simulink library "Capacitor"  (R2020b)
settings: Solver=ode45  StartTime=0.0  StopTime=10.0  RelTol=1e-3  EnableMultiTasking=on
undefined symbols (not defined in the file): Fsw_M, L_M, QgTotal_M, RL_M, Ron_M, Vgate_M
libraries: Lib_Dyn_StateSpace_TMATS x2, Lib_PF_BusLoadDC_TMATS x1
Description:
  | Thomas Modules
settings Model: Creator=jwchapm2  LastModifiedBy=nbutler2
settings DataIOCC: LimitDataPoints=on  SaveFormat=Array  ReturnWorkspaceOutputs=off
settings OptimizationCC: ExpressionDepthLimit=2147483647  LifeSpan=inf
settings DebuggingCC: UnderspecifiedInitializationDetection=Classic  MergeDetectMultiDrivingBlocksExec=none  SolverPrmCheckMsg=warning  StateNameClashWarn=warning  SFUnexpectedBacktrackingDiag=warning  SFNoUnconditionalDefaultTransitionDiag=warning  SFExecutionAtInitializationDiag=none  ArithmeticOperatorsInVariantConditions=warning
settings HardwareCC: ProdBitPerPointer=32  ProdBitPerSizeT=32  ProdBitPerPtrDiffT=32  ProdLargestAtomicFloat=None  ProdIntDivRoundTo=Undefined  ProdEndianess=Unspecified  ProdWordSize=32  ProdHWDeviceType=32-bit Generic
settings ModelReferenceCC: PropagateSignalLabelsOutOfModel=off
settings SFSimCC: SimUseLocalCustomCode=off  CustomCodeUndefinedFunction=UseInterfaceOnly
settings RTWCC: RTWUseLocalCustomCode=off
settings CodeAppCC: StateflowObjectComments=on
settings GRTTargetCC: TargetLangStandard=C89/C90 (ANSI)
settings ConfigComp: CovMetricSettings=dw  CovSaveCumulativeToWorkspaceVar=on  CovSaveSingleToWorkspaceVar=on  CovExternalEMLEnable=off

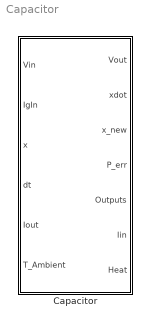
== system Capacitor ==
  Capacitor : Subsystem  mask(Capacitor){Pdis_M=1, C_M=600e-6, RC_M=1e-3, TempIn=Celsius}
      mask prompts: Pdis_M "Pdis_M - Constant Power Leaked/Dissipated, W"; C_M "C_M - Capacitor, Farads"; RC_M "RC_M - Resistance of Capacitor, Ohms"; TempIn "Input Temp Units"
      mask help: This block represents a generic capacitor energy storage element. The input current is solved for, such that the power in equals the power out.
      mask init:
      | %Get current block name
      | block = gcb;
      | 
      | %Block under the mask(T_in inport)
      | block2 = [block '/T_Ambient'];
      | 
      | %Set T_in unit parameter to correct unit.
      | switch TempIn
      |     case 1 
      |         set_param(block2,'Unit','degF');
      |     case 2
      |         set_param(block2,'Unit','degC');
      |     case 3
      |         set_param(block2,'Unit','degR');
      |     case 4
      |         set_param(block2,'Unit','K');
      | end
      mask TypeOptions TempIn: Fahrenheit | Celsius | Rankine | Kelvin
      mask DialogControl Container10 Prompt: Physical Parameters
      mask DialogControl Container11 Prompt: Temperature Units
      mask Display:
      | switch TempIn
      |     case 1
      |         port_label('input', 6, 'T_Ambient (F)');
      |     case 2
      |         port_label('input', 6, 'T_Ambient (C)');
      |     case 3
      |         port_label('input', 6, 'T_Ambient (Ra)');
      |     case 4
      |         port_label('input', 6, 'T_Ambient (K)');
      | end
      | 
      | port_label('input', 1, 'Vin');
      | port_label('input', 2, 'IgIn');
      | port_label('input', 3, 'x');
      | port_label('input', 4, 'dt');
      | port_label('input', 5, 'Idemand');
      | 
      | 
      | 
      | port_label('output', 1, 'Vout');
      | port_label('output', 2, 'xdot');
      | port_label('output', 3, 'x_new');
      | port_label('output', 4, 'P_err');
      | port_label('output', 5, 'Outputs');
      | port_label('output', 6, 'Idemanded');
      | port_label('output', 7, 'Heat');

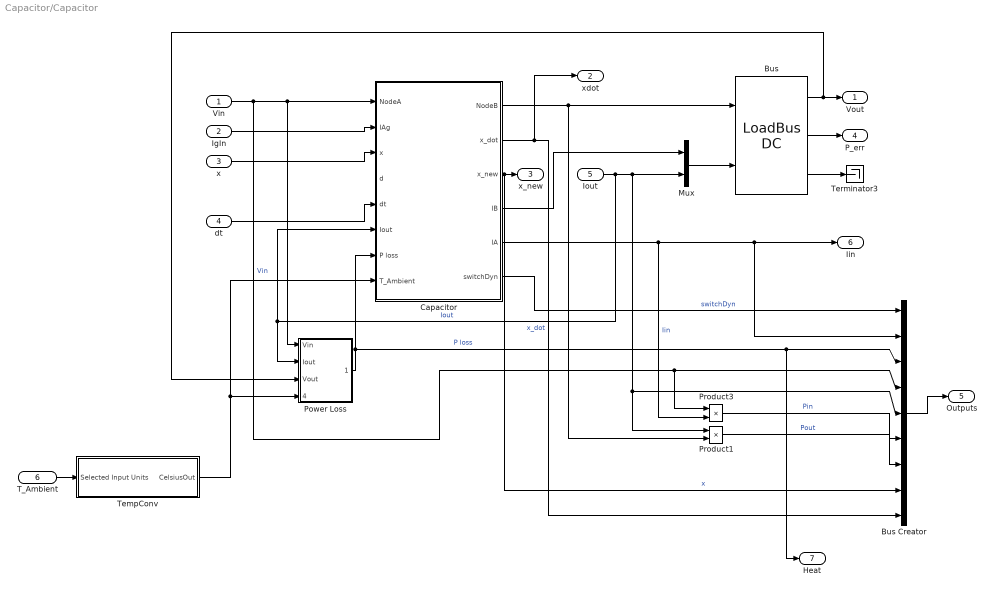
== system Capacitor/Capacitor ==
  Vin : Inport
  IgIn : Inport  Port=2
  x : Inport  Port=3
  dt : Inport  Port=4
  Iout : Inport  Port=5
  T_Ambient : Inport  Port=6  Unit=degC
  Bus : Lib_PF_BusLoadDC_TMATS/LoadBus DC  PeInEN_M=off  P_M=-Pdis_M  BlkNm_M=double(gcb)
  Bus Creator : BusCreator  Inputs=9
  Capacitor : Subsystem
      mask Display:
      | fprintf('Capacitor')
      | 
      | port_label('input',1,'VA')
      | port_label('input',2,'IAg')
      | port_label('input',3,'x')
      | port_label('input',4,'d')
      | port_label('input',5,'dt')
      | port_label('input',6,'Iout')
      | port_label('input',7,'Ploss')
      | 
      | 
      | port_label('output',1,'VB')
      | port_label('output',2,'x_dot')
      | port_label('output',3,'x_new')
      | port_label('output',4,'IB')
      | port_label('output',5,'IA')
      | port_label('output',6,'switchDyn')
  Mux : Mux  Inputs=2
  "Power Loss " : Subsystem
  Product1 : Product
  Product3 : Product
  "TempConv " : Subsystem  AncestorBlock=Lib_PB_MultiLevelInverter_TMATS/HiFiInverter/TempConv
      mask DialogControl DescTextVar Prompt: Temperature Unit Converter
  Terminator3 : Terminator
  Vout : Outport  VectorParamsAs1DForOutWhenUnconnected=off
  xdot : Outport  Port=2  VectorParamsAs1DForOutWhenUnconnected=off
  x_new : Outport  Port=3  VectorParamsAs1DForOutWhenUnconnected=off
  P_err : Outport  Port=4  VectorParamsAs1DForOutWhenUnconnected=off
  Outputs : Outport  Port=5  VectorParamsAs1DForOutWhenUnconnected=off
  Iin : Outport  Port=6  VectorParamsAs1DForOutWhenUnconnected=off
  Heat : Outport  Port=7  VectorParamsAs1DForOutWhenUnconnected=off
  wires:
  Bus Creator/1 -> Outputs/1
  Bus/2 -> P_err/1
  Bus/3 -> Terminator3/1
  Mux/1 -> Bus/2
  Capacitor/1(NodeB) -> Product1/2, Bus/1
  Vin/1 -> Capacitor/1(NodeA), "Power Loss "/1(Vin), Product3/1, Bus Creator/4  "Vin"
  Product3/1 -> Bus Creator/6  "Pin"
  Product1/1 -> Bus Creator/7  "Pout"
  Bus/1 -> Vout/1, "Power Loss "/3(Vout)
  Iout/1 -> Capacitor/6(Iout), "Power Loss "/2(Iout), Product1/1, Bus Creator/5, Mux/2  "Iout"
  Capacitor/2(x_dot) -> Bus Creator/9, xdot/1  "x_dot"
  Capacitor/4(IB) -> Mux/1
  Capacitor/5(IA) -> Product3/2, Bus Creator/2, Iin/1  "Iin"
  IgIn/1 -> Capacitor/2(IAg)
  x/1 -> Capacitor/3(x)
  "Power Loss "/1(" P loss") -> Capacitor/7(P loss), Heat/1, Bus Creator/3  "P loss"
  Capacitor/3(x_new) -> Bus Creator/8, x_new/1  "x"
  dt/1 -> Capacitor/5(dt)
  Capacitor/6(switchDyn) -> Bus Creator/1  "switchDyn"
  T_Ambient/1 -> "TempConv "/1(Selected Input Units)
  "TempConv "/1(CelsiusOut) -> "Power Loss "/4("T_Ambient "), Capacitor/8("T_Ambient ")

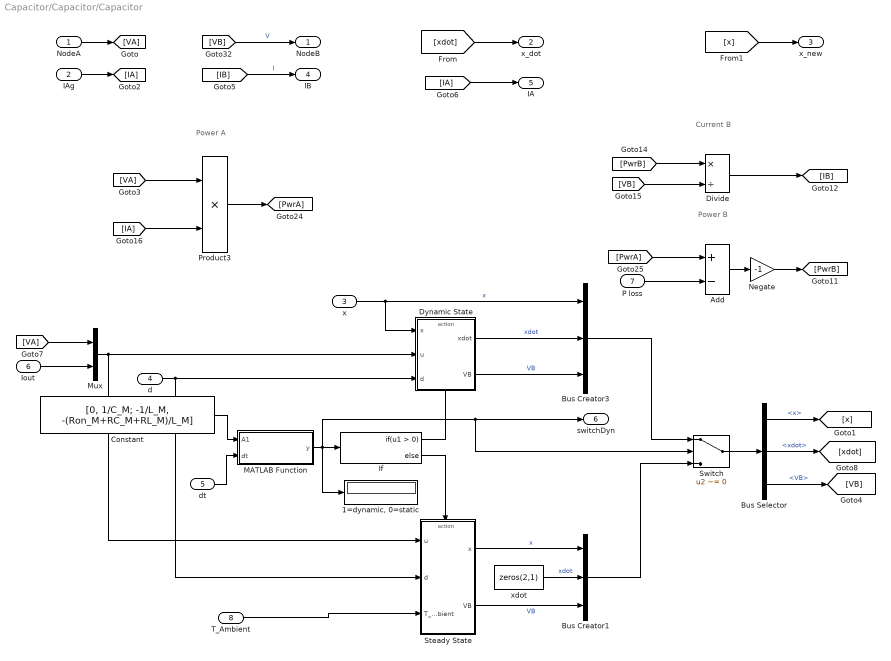
== system Capacitor/Capacitor/Capacitor ==
  note: Power A
  note: Current B
  note: Power B
  NodeA : Inport
  IAg : Inport  Port=2
  x : Inport  Port=3
  d : Inport  Port=4
  dt : Inport  Port=5
  Iout : Inport  Port=6
  P loss : Inport  Port=7
  "T_Ambient " : Inport  Port=8
  " Dynamic State" : Subsystem  TreatAsAtomicUnit=on
  "1=dynamic, 0=static" : Display
  Add : Sum  Inputs=+-
  Bus Creator1 : BusCreator  Inputs=3
  Bus Creator3 : BusCreator  Inputs=3
  Bus Selector : BusSelector  OutputSignals=x,xdot,VB
  Constant : Constant  Value=[0, 1/C_M; -1/L_M, -(Ron_M+RC_M+RL_M)/L_M]  VectorParams1D=off
  Divide : Product  Inputs=*/
  If : If
  MATLAB Function : MATLAB Function  TreatAsAtomicUnit=on
  Mux : Mux  Inputs=2
  Negate : Gain  Gain=-1
  Product3 : Product
  Steady State : Subsystem  TreatAsAtomicUnit=on
  Switch : Switch  Criteria=u2 ~= 0
  xdot : Constant  Value=zeros(2,1)  VectorParams1D=off
  NodeB : Outport  VectorParamsAs1DForOutWhenUnconnected=off
  x_dot : Outport  Port=2  VectorParamsAs1DForOutWhenUnconnected=off
  x_new : Outport  Port=3  VectorParamsAs1DForOutWhenUnconnected=off
  IB : Outport  Port=4  VectorParamsAs1DForOutWhenUnconnected=off
  IA : Outport  Port=5  VectorParamsAs1DForOutWhenUnconnected=off
  switchDyn : Outport  Port=6  VectorParamsAs1DForOutWhenUnconnected=off
  wires:
  Bus Creator1/1 -> Switch/3
  [VA] -> Product3/1
  Product3/1 -> [PwrA]
  [VB] -> NodeB/1  "V"
  NodeA/1 -> [VA]
  [IA] -> Product3/2
  [PwrB] -> Divide/1
  Divide/1 -> [IB]
  [VB] -> Divide/2
  IAg/1 -> [IA]
  [IB] -> IB/1  "I"
  [IA] -> IA/1
  MATLAB Function/1(y) -> "1=dynamic, 0=static"/1, Switch/2, switchDyn/1, If/1
  If/1 -> " Dynamic State"/Action
  Constant/1 -> MATLAB Function/1(A1)
  If/2 -> Steady State/Action
  dt/1 -> MATLAB Function/2(dt)
  Steady State/1(x) -> Bus Creator1/1  "x"
  x/1 -> Bus Creator3/1, " Dynamic State"/1(x)  "x"
  d/1 -> Steady State/2(d), " Dynamic State"/3(d)
  [xdot] -> x_dot/1
  [PwrA] -> Add/1
  P loss/1 -> Add/2
  Add/1 -> Negate/1
  Switch/1 -> Bus Selector/1
  " Dynamic State"/2(VB) -> Bus Creator3/3  "VB"
  " Dynamic State"/1(xdot) -> Bus Creator3/2  "xdot"
  Steady State/2(VB) -> Bus Creator1/3  "VB"
  xdot/1 -> Bus Creator1/2  "xdot"
  Bus Selector/3 -> [VB]  "<VB>"
  Bus Selector/2 -> [xdot]  "<xdot>"
  Bus Selector/1 -> [x]  "<x>"
  Bus Creator3/1 -> Switch/1
  [x] -> x_new/1
  [VA] -> Mux/1
  Iout/1 -> Mux/2
  Mux/1 -> Steady State/1(u), " Dynamic State"/2(u)
  Negate/1 -> [PwrB]
  "T_Ambient "/1 -> Steady State/3("T_Ambient ")

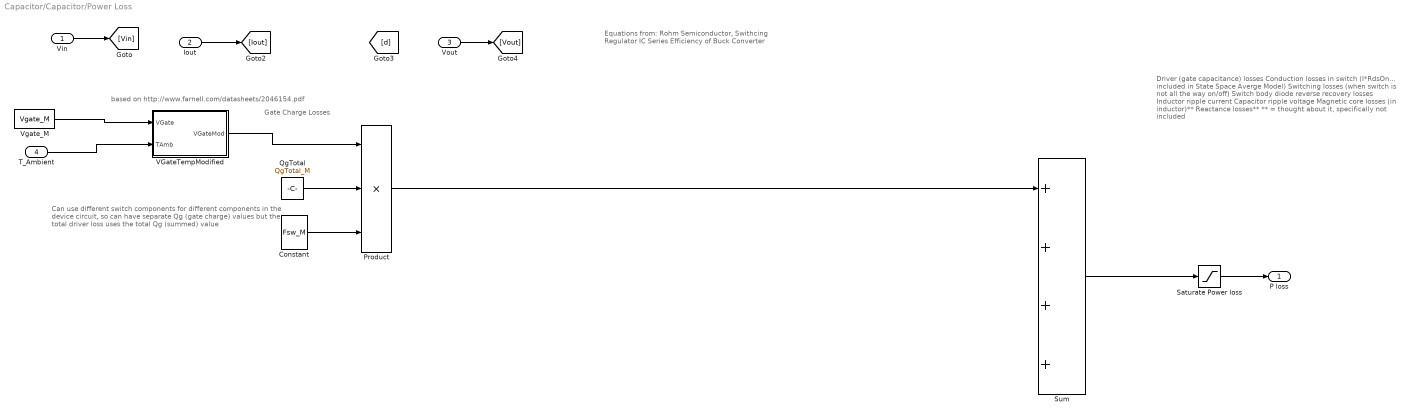
== system Capacitor/Capacitor/Power Loss  ==
  note: Equations from:
      | Rohm Semiconductor, Swithcing Regulator IC Series
      | Efficiency of Buck Converter
  note: Gate Charge Losses
  note: Can use different switch components for different components in
      | the device circuit, so can have separate Qg (gate charge) values
      | but the total driver loss uses the total Qg (summed) value
  note: Driver (gate capacitance) losses
      | Conduction losses in switch (I*RdsOn... included in State Space Averge Model)
      | Switching losses (when switch is not all the way on/off)
      | Switch body diode reverse recovery losses
      | Inductor ripple current
      | Capacitor ripple voltage
      | Magnetic core losses (in inductor)**
      | Reactance losses**
      | ** = thought about it, specifically not included
  note: based on http://www.farnell.com/datasheets/2046154.pdf
  Vin : Inport
  Iout : Inport  Port=2
  Vout : Inport  Port=3
  "T_Ambient " : Inport  Port=4
  Constant : Constant  Value=Fsw_M
  Product : Product  Inputs=3
  QgTotal : Constant  Value=QgTotal_M  VectorParams1D=off
  Saturate Power loss : Saturate  UpperLimit=inf  LowerLimit=0
  Sum : Sum  Inputs=++++
  VGateTempModified : Subsystem  AncestorBlock=Lib_PFSys_HiFiBoostConv_TMATS_Thermal/Boost Converter/Power Loss /VGateTempModified
  Vgate_M : Constant  Value=Vgate_M
  " P loss" : Outport  VectorParamsAs1DForOutWhenUnconnected=off
  wires:
  Product/1 -> Sum/1
  QgTotal/1 -> Product/2
  Saturate Power loss/1 -> " P loss"/1
  Sum/1 -> Saturate Power loss/1
  Vin/1 -> [Vin]
  Iout/1 -> [Iout]
  ? -> [d]
  Vout/1 -> [Vout]
  Constant/1 -> Product/3
  Vgate_M/1 -> VGateTempModified/1("VGate ")
  "T_Ambient "/1 -> VGateTempModified/2(TAmb)
  VGateTempModified/1("VGateMod ") -> Product/1

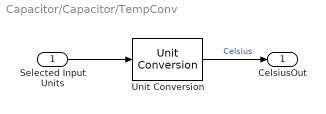
== system Capacitor/Capacitor/TempConv  ==
  Selected Input Units : Inport
  Unit Conversion : UnitConversion
  CelsiusOut : Outport  Unit=°C  VectorParamsAs1DForOutWhenUnconnected=off
  wires:
  Selected Input Units/1 -> Unit Conversion/1
  Unit Conversion/1 -> CelsiusOut/1  "Celsius"

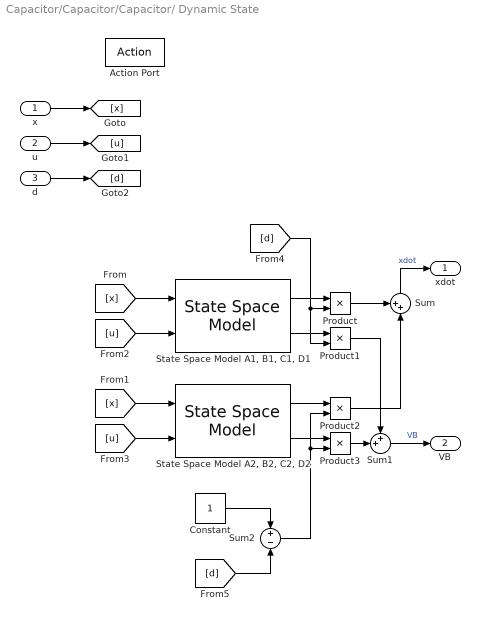
== system Capacitor/Capacitor/Capacitor/ Dynamic State ==
  x : Inport
  u : Inport  Port=2
  d : Inport  Port=3
  Action Port : ActionPort
  Constant : Constant
  Product{,1..3} (4 alike) : Product
  "State Space Model A1, B1, C1, D1" : Lib_Dyn_StateSpace_TMATS/State Space Model  A_M=[0, 1/C_M; -1/L_M, -(Ron_M+RC_M+RL_M)/L_M]  B_M=[0, -1/C_M; 1/L_M, RC_M/L_M]  C_M="[1,  RC_M]"  D_M=[0, -RC_M]
  "State Space Model A2, B2, C2, D2" : Lib_Dyn_StateSpace_TMATS/State Space Model  A_M=[0, 1/C_M; -1/L_M, -(Ron_M+RC_M+RL_M)/L_M]  B_M=[0, -1/C_M; 0, RC_M/L_M]  C_M="[1,  RC_M]"  D_M=[0, -RC_M]
  Sum : Sum  Inputs=++|
  Sum1 : Sum  Inputs=++|
  Sum2 : Sum  Inputs=+-
  xdot : Outport  VectorParamsAs1DForOutWhenUnconnected=off
  VB : Outport  Port=2  VectorParamsAs1DForOutWhenUnconnected=off
  wires:
  Sum/1 -> xdot/1  "xdot"
  Sum1/1 -> VB/1  "VB"
  Product/1 -> Sum/1
  Product1/1 -> Sum1/1
  x/1 -> [x]
  Product2/1 -> Sum/2
  "State Space Model A2, B2, C2, D2"/1 -> Product2/1
  "State Space Model A2, B2, C2, D2"/2 -> Product3/1
  Product3/1 -> Sum1/2
  [u] -> "State Space Model A2, B2, C2, D2"/2
  [x] -> "State Space Model A2, B2, C2, D2"/1
  u/1 -> [u]
  [d] -> Sum2/2
  [d] -> Product/2, Product1/2
  [u] -> "State Space Model A1, B1, C1, D1"/2
  "State Space Model A1, B1, C1, D1"/2 -> Product1/1
  [x] -> "State Space Model A1, B1, C1, D1"/1
  Constant/1 -> Sum2/1
  Sum2/1 -> Product3/2, Product2/2
  d/1 -> [d]
  "State Space Model A1, B1, C1, D1"/1 -> Product/1

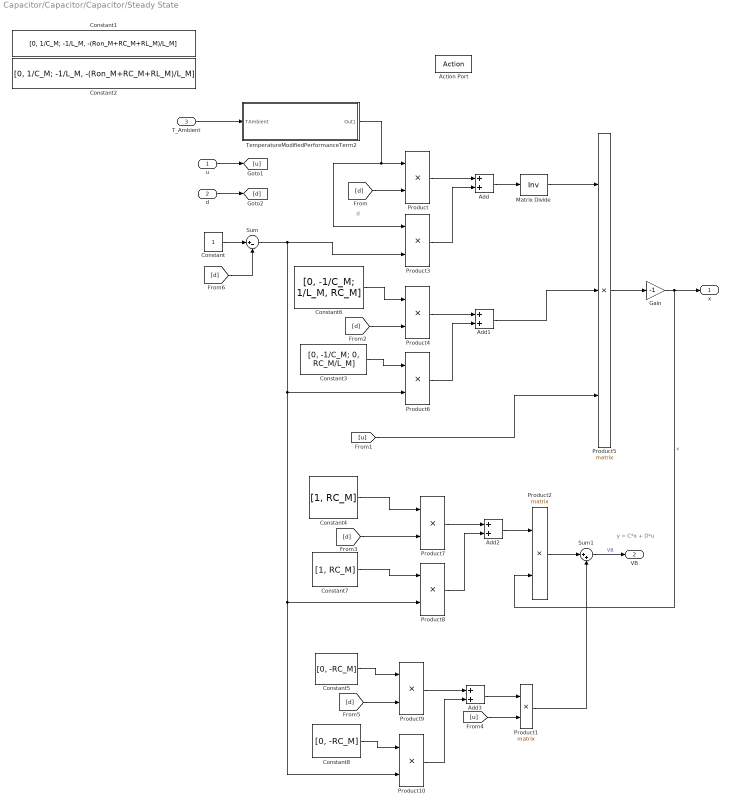
== system Capacitor/Capacitor/Capacitor/Steady State ==
  note: y = C*x + D*u
  note: d
  u : Inport
  d : Inport  Port=2
  "T_Ambient " : Inport  Port=3
  Action Port : ActionPort
  Add{,1..3} (4 alike) : Sum
  Constant : Constant
  Constant1 : Constant  Value=[0, 1/C_M; -1/L_M, -(Ron_M+RC_M+RL_M)/L_M]  VectorParams1D=off
  Constant2 : Constant  Value=[0, 1/C_M; -1/L_M, -(Ron_M+RC_M+RL_M)/L_M]  VectorParams1D=off
  Constant3 : Constant  Value=[0, -1/C_M; 0, RC_M/L_M]  VectorParams1D=off
  Constant4 : Constant  Value=[1, RC_M]  VectorParams1D=off
  Constant5 : Constant  Value=[0, -RC_M]  VectorParams1D=off
  Constant6 : Constant  Value=[0, -1/C_M; 1/L_M, RC_M]  VectorParams1D=off
  Constant7 : Constant  Value=[1, RC_M]  VectorParams1D=off
  Constant8 : Constant  Value=[0, -RC_M]  VectorParams1D=off
  Gain : Gain  Gain=-1
  Matrix Divide : Product  Inputs=/  Multiplication=Matrix(*)
  Product{,3..4,6..10} (8 alike) : Product
  Product1 : Product  Multiplication=Matrix(*)
  Product2 : Product  Multiplication=Matrix(*)
  Product5 : Product  Inputs=3  Multiplication=Matrix(*)
  Sum : Sum  Inputs=|+-
  Sum1 : Sum  Inputs=|++
  "TemperatureModifiedPerformanceTerm2 " : Subsystem  AncestorBlock=Lib_PFSys_HiFiBoostConv_TMATS_Thermal/Boost Converter/DC - DC Converter/Steady State/TemperatureModifiedPerformanceTerm2
  x : Outport  VectorParamsAs1DForOutWhenUnconnected=off
  VB : Outport  Port=2  VectorParamsAs1DForOutWhenUnconnected=off
  wires:
  [u] -> Product1/2
  Add2/1 -> Product2/1
  Product9/1 -> Add3/1
  Matrix Divide/1 -> Product5/1
  Product3/1 -> Add/2
  Constant3/1 -> Product6/1
  Product/1 -> Add/1
  [d] -> Product9/2
  Product4/1 -> Add1/1
  Sum1/1 -> VB/1  "VB"
  Product7/1 -> Add2/1
  d/1 -> [d]
  Product2/1 -> Sum1/1
  u/1 -> [u]
  Constant4/1 -> Product7/1
  Gain/1 -> Product2/2, x/1  "x"
  [d] -> Product4/2
  [u] -> Product5/3
  Constant6/1 -> Product4/1
  Constant/1 -> Sum/1
  Add3/1 -> Product1/1
  Sum/1 -> Product3/2, Product6/2, Product8/2, Product10/2
  Product5/1 -> Gain/1
  Product1/1 -> Sum1/2
  [d] -> Sum/2
  Constant5/1 -> Product9/1
  [d] -> Product/2
  Product10/1 -> Add3/2
  Product8/1 -> Add2/2
  Add1/1 -> Product5/2
  [d] -> Product7/2
  Constant7/1 -> Product8/1
  Add/1 -> Matrix Divide/1
  Product6/1 -> Add1/2
  Constant8/1 -> Product10/1
  "TemperatureModifiedPerformanceTerm2 "/1(Out1) -> Product/1, Product3/1
  "T_Ambient "/1 -> "TemperatureModifiedPerformanceTerm2 "/1(TAmbient)

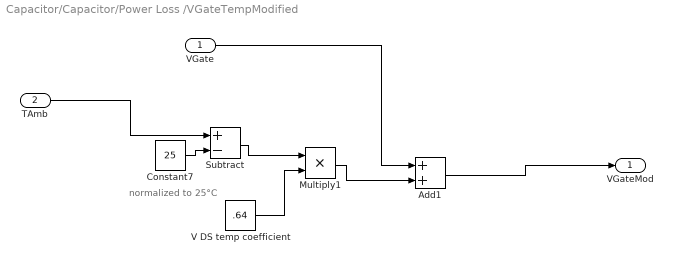
== system Capacitor/Capacitor/Power Loss /VGateTempModified ==
  note: normalized to 25°C
  "VGate " : Inport
  TAmb : Inport  Port=2
  Add1 : Sum
  Constant7 : Constant  Value=25
  Multiply1 : Product
  Subtract : Sum  Inputs=+-
  "V DS temp coefficient " : Constant  Value=.64
  "VGateMod " : Outport  VectorParamsAs1DForOutWhenUnconnected=off
  wires:
  Multiply1/1 -> Add1/2
  Constant7/1 -> Subtract/2
  "VGate "/1 -> Add1/1
  TAmb/1 -> Subtract/1
  Subtract/1 -> Multiply1/1
  "V DS temp coefficient "/1 -> Multiply1/2
  Add1/1 -> "VGateMod "/1

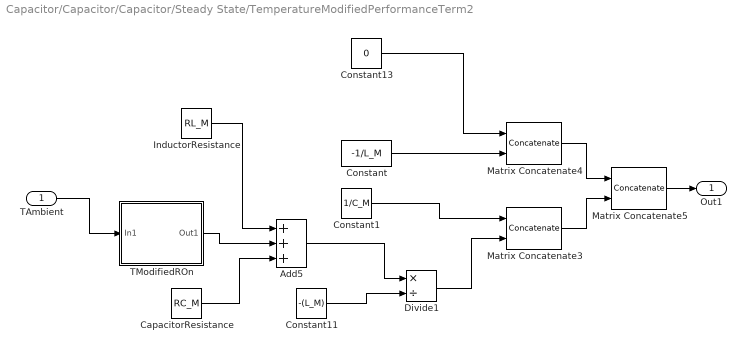
== system Capacitor/Capacitor/Capacitor/Steady State/TemperatureModifiedPerformanceTerm2  ==
  TAmbient : Inport
  Add5 : Sum  Inputs=+++
  CapacitorResistance : Constant  Value=RC_M
  Constant : Constant  Value=-1/L_M
  Constant1 : Constant  Value=1/C_M
  Constant11 : Constant  Value=-(L_M)
  Constant13 : Constant  Value=0
  Divide1 : Product  Inputs=*/
  "InductorResistance " : Constant  Value=RL_M
  Matrix Concatenate3 : Concatenate  Mode=Multidimensional array
  Matrix Concatenate4 : Concatenate  Mode=Multidimensional array
  Matrix Concatenate5 : Concatenate  Mode=Multidimensional array  ConcatenateDimension=2
  "TModifiedROn " : Subsystem
  Out1 : Outport  VectorParamsAs1DForOutWhenUnconnected=off
  wires:
  Constant11/1 -> Divide1/2
  Add5/1 -> Divide1/1
  Matrix Concatenate3/1 -> Matrix Concatenate5/2
  Divide1/1 -> Matrix Concatenate3/2
  Matrix Concatenate4/1 -> Matrix Concatenate5/1
  Constant13/1 -> Matrix Concatenate4/1
  "TModifiedROn "/1(Out1) -> Add5/2
  "InductorResistance "/1 -> Add5/1
  TAmbient/1 -> "TModifiedROn "/1(In1)
  Matrix Concatenate5/1 -> Out1/1
  CapacitorResistance/1 -> Add5/3
  Constant1/1 -> Matrix Concatenate3/1
  Constant/1 -> Matrix Concatenate4/2

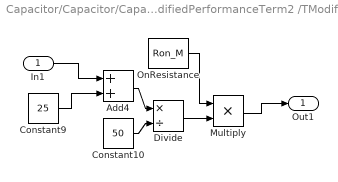
== system Capacitor/Capacitor/Capacitor/Steady State/TemperatureModifiedPerformanceTerm2 /TModifiedROn  ==
  In1 : Inport
  Add4 : Sum
  Constant10 : Constant  Value=50
  Constant9 : Constant  Value=25
  Divide : Product  Inputs=*/
  Multiply : Product
  "OnResistance " : Constant  Value=Ron_M
  Out1 : Outport  VectorParamsAs1DForOutWhenUnconnected=off
  wires:
  "OnResistance "/1 -> Multiply/1
  Multiply/1 -> Out1/1
  Divide/1 -> Multiply/2
  Constant9/1 -> Add4/2
  Add4/1 -> Divide/1
  Constant10/1 -> Divide/2
  In1/1 -> Add4/1

== matlab function Capacitor/Capacitor/MATLAB Function ==
  data: A1 input; y output; dt input
function y  = switchLogic(A1, dt)    %A1 state martix, dt time step    

StableFlag=all(abs(1+dt*eig(A1))<=1);    %Forward Euler Stability requirement

if StableFlag==1
    y=1;    %runs dynamic model
    
else
    y=0;    %runs steady state model
    
end

end
